simulink subsystem "BLDC"  (R2022b)
settings: Solver=VariableStepAuto  StartTime=0.0  StopTime=10.0  RelTol=1e-3
values from neighbouring files (symbols this model uses):
  A = diag([-Rm/Lm -Rm/Lm])    [BLDCmotor.m]    (also in function_A_hover.m = reshape([0.0,t52,t52,t11.*t50,0.0,t46,t46,-t48,0.0,t47,t47,t; geraModeloHover.m = subs(A_sym))
  B = [ 2/(3*Lm) 1/(3*Lm) ... (first row only)    [BLDCmotor.m]    (also in function_B_hover.m = reshape([0.0,(t6.*t7.*t10.*t27.*t33.*t34)./2.0,(t6.*t7.*t10.; geraModeloHover.m = subs(B_sym))
  C = [ 1  0 ... (first row only)    [BLDCmotor.m]
  D = zeros(size(C, 1), size(B, 2))    [BLDCmotor.m]
  Ke = motor.Ke    [BLDCmotor.m]    (also in geraModeloHover.m = 0.509462836178)
  Kt = motor.Kt    [BLDCmotor.m]    (also in geraModeloHover.m = 0.999243570348)
  p = motor.p    [BLDCmotor.m]    (also in geraModeloHover.m = 30)
settings Model: Creator=hemil  LastModifiedBy=hemil
settings OptimizationCC: ReuseModelBlockBuffer=on

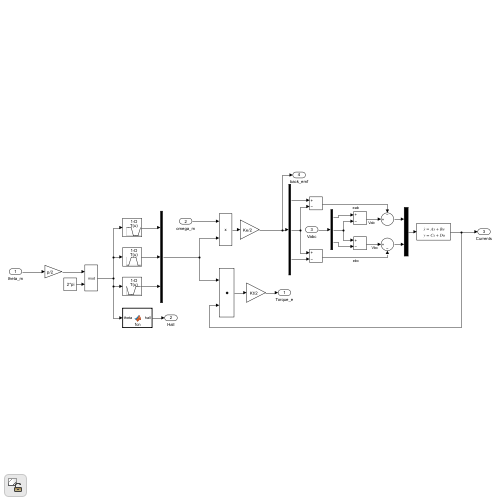
[thumbnail: Simulink's stored preview of the top-level diagram]
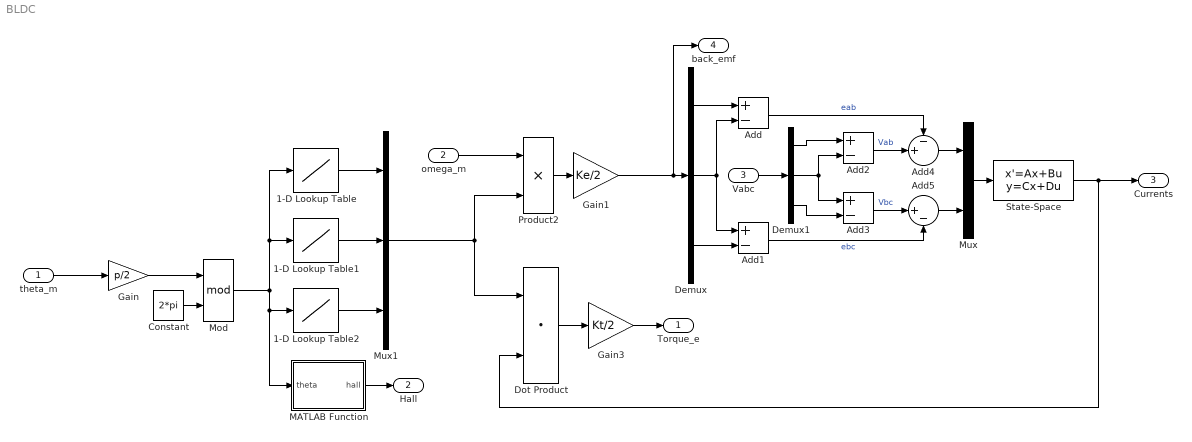
== system BLDC ==
  theta_m : Inport
  omega_m : Inport  Port=2
  Vabc : Inport  Port=3
  1-D Lookup Table : Lookup_n-D  NumberOfTableDimensions=1  BreakpointsSpecification=Even spacing  BreakpointsForDimension1=[0 pi/3 2*pi/3 pi 4*pi/3 5*pi/3 2*pi]  BreakpointsForDimension1FirstPoint=0  BreakpointsForDimension1Spacing=pi/3  Table=[1 1 1 -1 -1 -1 1]  InternalRulePriority=Speed  RndMeth=Simplest
  1-D Lookup Table1 : Lookup_n-D  NumberOfTableDimensions=1  BreakpointsSpecification=Even spacing  BreakpointsForDimension1=[0 pi/3 2*pi/3 pi 4*pi/3 5*pi/3 2*pi]  BreakpointsForDimension1FirstPoint=0  BreakpointsForDimension1Spacing=pi/3  Table=[-1 -1 1 1 1 -1 -1]  InternalRulePriority=Speed  RndMeth=Simplest
  1-D Lookup Table2 : Lookup_n-D  NumberOfTableDimensions=1  BreakpointsSpecification=Even spacing  BreakpointsForDimension1=[0 pi/3 2*pi/3 pi 4*pi/3 5*pi/3 2*pi]  BreakpointsForDimension1FirstPoint=0  BreakpointsForDimension1Spacing=pi/3  Table=[1 -1 -1 -1 1 1 1]  InternalRulePriority=Speed  RndMeth=Simplest
  Add{,1..3} (4 alike) : Sum  Inputs=+-
  Add4 : Sum  Inputs=-+|
  Add5 : Sum  Inputs=|+-
  Constant : Constant  Value=2*pi
  Demux : Demux  Outputs=3
  Demux1 : Demux  Outputs=3
  Dot Product : DotProduct  OutDataTypeStr=Inherit: Inherit via internal rule
  Gain : Gain  Gain=p/2
  Gain1 : Gain  Gain=Ke/2
  Gain3 : Gain  Gain=Kt/2
  MATLAB Function : MATLAB Function  TreatAsAtomicUnit=on
  Mod : Math  Operator=mod
  Mux : Mux  Inputs=2
  Mux1 : Mux  Inputs=3
  Product2 : Product
  State-Space : StateSpace  A=A  B=B  C=C  D=D  InitialCondition=0
  Torque_e : Outport
  Hall : Outport  Port=2
  Currents : Outport  Port=3
  back_emf : Outport  Port=4
  wires:
  Product2/1 -> Gain1/1
  1-D Lookup Table2/1 -> Mux1/3
  1-D Lookup Table1/1 -> Mux1/2
  Mod/1 -> 1-D Lookup Table/1, 1-D Lookup Table1/1, 1-D Lookup Table2/1, MATLAB Function/1(theta)
  1-D Lookup Table/1 -> Mux1/1
  theta_m/1 -> Gain/1
  omega_m/1 -> Product2/1
  Dot Product/1 -> Gain3/1
  Mux1/1 -> Dot Product/1, Product2/2
  Gain3/1 -> Torque_e/1
  State-Space/1 -> Dot Product/2, Currents/1
  MATLAB Function/1(hall) -> Hall/1
  Demux/1 -> Add/1
  Demux/2 -> Add1/1, Add/2
  Demux/3 -> Add1/2
  Add/1 -> Add4/1  "eab"
  Mux/1 -> State-Space/1
  Add4/1 -> Mux/1
  Add5/1 -> Mux/2
  Add1/1 -> Add5/2  "ebc"
  Vabc/1 -> Demux1/1
  Demux1/1 -> Add2/1
  Demux1/2 -> Add2/2, Add3/1
  Demux1/3 -> Add3/2
  Add3/1 -> Add5/1  "Vbc"
  Add2/1 -> Add4/2  "Vab"
  Gain1/1 -> Demux/1, back_emf/1
  Gain/1 -> Mod/1
  Constant/1 -> Mod/2

== matlab function BLDC/MATLAB Function ==
  data: theta input; hall output
function hall = fcn(theta)
    hall = zeros(3, 1);
    if theta < pi/3 % 100
        hall(1) = 1;
    elseif theta < 2*pi/3 % 110
        hall(1) = 1;
        hall(2) = 1;
    elseif theta < pi % 010
        hall(2) = 1;
    elseif theta < 4*pi/3 % 011
        hall(2) = 1;
        hall(3) = 1;
    elseif theta < 5*pi/3 % 001
        hall(3) = 1;
    else % 101
        hall(1) = 1;
        hall(3) = 1;
    end
